simulink model "Ej_3_1_m3"  (R2022b)
settings: Solver=VariableStepAuto  StartTime=0.0  StopTime=40  RelTol=1e-3
settings Model: Creator=rrilo  LastModifiedBy=rrilo

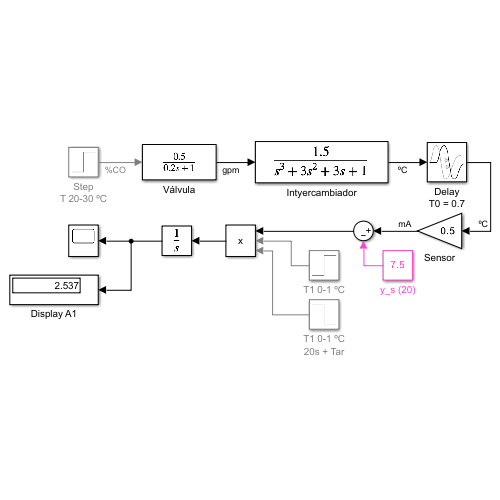
[thumbnail: Simulink's stored preview of the top-level diagram]
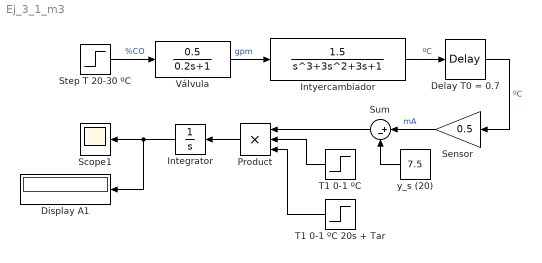
== system Ej_3_1_m3 ==
  Delay T0 = 0.7 : TransportDelay  DelayTime=0.7
  Display A1 : Display
  Integrator : Integrator
  Intyercambiador : TransferFcn  Numerator=[1.5]  Denominator=[1 3 3 1]
  Product : Product  Inputs=3
  Scope1 : Scope
  Sensor : Gain  Gain=0.5
  Step T 20-30 ºC : Step  Time=20  Before=20  After=30  SampleTime=0
  Sum : Sum  Inputs=|+-
  T1 0-1 ºC : Step  Time=20  SampleTime=0
  T1 0-1 ºC 20s + Tar : Step  Time=20+3.9  Before=1  After=0  SampleTime=0
  Válvula : TransferFcn  Numerator=[0.5]  Denominator=[0.2 1]
  y_s (20) : Constant  Value=7.5
  wires:
  Sensor/1 -> Sum/1  "mA"
  Intyercambiador/1 -> Delay T0 = 0.7/1  "ºC"
  Step T 20-30 ºC/1 -> Válvula/1  "%CO"
  Válvula/1 -> Intyercambiador/1  "gpm"
  Delay T0 = 0.7/1 -> Sensor/1  "ºC"
  y_s (20)/1 -> Sum/2
  Integrator/1 -> Display A1/1, Scope1/1
  Product/1 -> Integrator/1
  T1 0-1 ºC/1 -> Product/2
  Sum/1 -> Product/1
  T1 0-1 ºC 20s + Tar/1 -> Product/3
